simulink library "findEulerAngles_ul"  (R2018a)
settings: Solver=VariableStepAuto  StartTime=0.0  StopTime=10.0  RelTol=1e-3
settings Model: Creator=mcobb  LastModifiedBy=mcobb

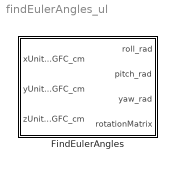
== system findEulerAngles_ul ==
  FindEulerAngles : Subsystem

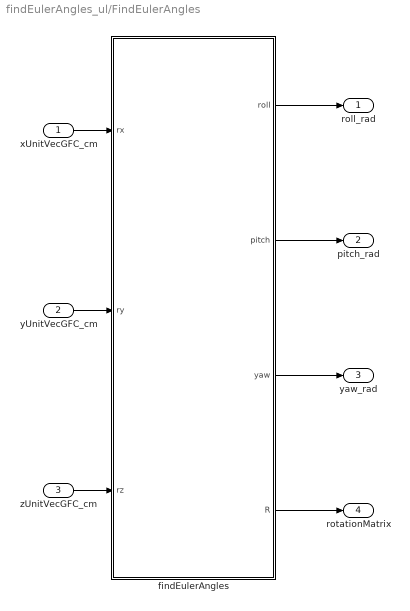
== system findEulerAngles_ul/FindEulerAngles ==
  xUnitVecGFC_cm : Inport
  yUnitVecGFC_cm : Inport  Port=2
  zUnitVecGFC_cm : Inport  Port=3
  findEulerAngles : MATLAB Function  TreatAsAtomicUnit=on
  roll_rad : Outport
  pitch_rad : Outport  Port=2
  yaw_rad : Outport  Port=3
  rotationMatrix : Outport  Port=4
  wires:
  xUnitVecGFC_cm/1 -> findEulerAngles/1(rx)
  yUnitVecGFC_cm/1 -> findEulerAngles/2(ry)
  zUnitVecGFC_cm/1 -> findEulerAngles/3(rz)
  findEulerAngles/1(roll) -> roll_rad/1
  findEulerAngles/2(pitch) -> pitch_rad/1
  findEulerAngles/3(yaw) -> yaw_rad/1
  findEulerAngles/4(R) -> rotationMatrix/1

== matlab function findEulerAngles_ul/FindEulerAngles/findEulerAngles ==
  data: rx input; ry input; rz input; roll output; pitch output; yaw output; R output
function [roll,pitch,yaw,R] = fcn(rx,ry,rz)
%#codegen
[roll,pitch,yaw,R] = findEulerAngles(rx,ry,rz);
end
